simulink model "simu"  (R2019b)
settings: Solver=VariableStepAuto  StartTime=0.0  StopTime=25.0  RelTol=1e-3
values from neighbouring files (symbols this model uses):
  k = b    (= 5)    [2ndSimulationProjectmain.m]
  rt = a    (= 10)    [2ndSimulationProjectmain.m]
  ut = a/2    (= 5)    [2ndSimulationProjectmain.m]
libraries: cstblocks x2
settings Model: Creator=Dell  LastModifiedBy=Dell

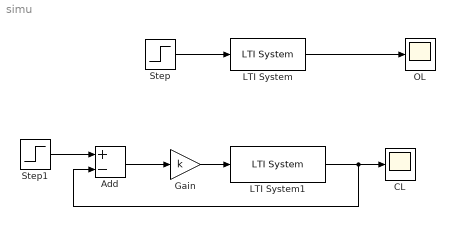
== system simu ==
  Add : Sum  Inputs=+-
  CL : Scope
  Gain : Gain  Gain=k
  LTI System : cstblocks/LTI System  sys=G2  IC=[]
  LTI System1 : cstblocks/LTI System  sys=G2  IC=[]
  OL : Scope
  Step : Step  Time=0  After=ut  SampleTime=0
  Step1 : Step  Time=0  After=rt  SampleTime=0
  wires:
  Step/1 -> LTI System/1
  LTI System/1 -> OL/1
  LTI System1/1 -> Add/2, CL/1
  Step1/1 -> Add/1
  Add/1 -> Gain/1
  Gain/1 -> LTI System1/1
